simulink model "BPM_HA_Spin_sfun_16k"  (R2018a)
settings: configuration reference "ModelConfig_var" (kept outside this file)
InitFcn:
  | %% BUS initialization
  | Xabc.A = 0;
  | Xabc.B = 0;
  | Xabc.C = 0;
  | % -------------------------------------------------------------------------
  | Simulink.Bus.createObject(Xabc)
  | XabcBus = slBus1;
  | clear slBus1
  | 
  | %% Parameter Structure initialization
  | Motor_prm_init_bpm;
model workspace (MAT data in the model file):
  Mech_HAs_CF = 0
  Mech_HAs_J_drum = 0
  Mech_HAs_TR = 0
  Mech_HAs_damp = 0
  Mech_HAs_m_unb = 0
  Mech_HAs_r_unb = 0
  Mech_VAa_J_basket = 0
  Mech_VAa_J_impeller = 0
  Mech_VAa_basket_dens = 0
  Mech_VAa_basket_dia = 0
  Mech_VAa_belt_ratio = 0
  Mech_VAa_clothes_mass = 0
  Mech_VAa_gear_ratio = 0
  Mech_VAa_imp_dens = 0
  Mech_VAa_water_vol = 0
  Mech_VAs_D_r = 0
  Mech_VAs_I_zt = 0
  Mech_VAs_K = 2700
  Mech_VAs_T_f = 0
  Mech_VAs_belt_rat = 0
  Mech_VAs_d = 0
  Mech_VAs_e = 0
  Mech_VAs_m_b1 = 0
  Mech_VAs_m_b2 = 0
  Mech_VAs_m_d = 0
  Mech_VAs_m_t = 0
  Mech_VAs_m_u = 0
  Time_step = 6.25e-05
  bpm_B = 0
  bpm_Ipk = [0 1 2 3 4 5 6 7]
  bpm_Jrotor = 0
  bpm_Ld_0 = 0.02117
  bpm_Ld_a = [0.02117 0.02117 0.02117 0.02117 0.02117 0.02117 0.02117 0.02117]
  bpm_Ldq_sat_flag = 0
  bpm_Loss_Power = [0 1 2 3 4 5 6 7]
  bpm_Loss_Speed = [0 1 2 3 4 5 6 7]
  bpm_Loss_flag = 0
  bpm_Loss_th = 5
  bpm_Lq_0 = 0.02117
  bpm_Lq_b = [0.02117 0.02117 0.02117 0.02117 0.02117 0.02117 0.02117 0.02117]
  bpm_NPP = 0
  bpm_PM_flux_h1_0 = 0
  bpm_PM_rotor_alpha = 0
  bpm_Rs_0 = 0
  bpm_Rs_stator_alpha = 0
  bpm_TR = 1
  bpm_Temp_rotor_0 = 0
  bpm_Temp_stator_0 = 0
libraries: bpm_dq_S_noH_D_RL_HA_Spin_16k x1
settings Model: ParameterArgumentNames=Mech_HAs_CF,Mech_HAs_J_drum,Mech_HAs_TR,Mech_HAs_damp,Mech_HAs_m_unb,Mech_HAs_r_unb,Mech_VAa_J_basket,Mech_VAa_J_impeller,Mech_VAa_basket_dens,Mech_VAa_basket_dia,Mech_VAa_belt_ratio,Mech_VAa_clothes_mass,Mech_VAa_gear_ratio,Mech_VAa_imp_dens,Mech_VAa_water_vol,Mech_VAs_D_r,Mech_VAs_I_zt,Mech_VAs_K,Mech_VAs_T_f,Mech_VAs_belt_rat,Mech_VAs_d,Mech_VAs_e,Mech_VAs_m_b1,Mech_VAs_m_b2,Mech_VAs_m_d,Mech_VAs_m_t,Mech_VAs_m_u,Time_step,bpm_B,bpm_Ipk,bpm_Jrotor,bpm_Ld_0,bpm_Ld_a,bpm_Ldq_sat_flag,bpm_Loss_Power,bpm_Loss_Speed,bpm_Loss_flag,bpm_Loss_th,bpm_Lq_0,bpm_Lq_b,bpm_NPP,bpm_PM_flux_h1_0,bpm_PM_rotor_alpha,bpm_Rs_0,bpm_Rs_stator_alpha,bpm_TR,bpm_Temp_rotor_0,bpm_Temp_stator_0  OrderedModelArguments=off  Creator=BEDNASA  LastModifiedBy=BEDNASA
settings ConfigSetRef: SourceLocation=Base Workspace

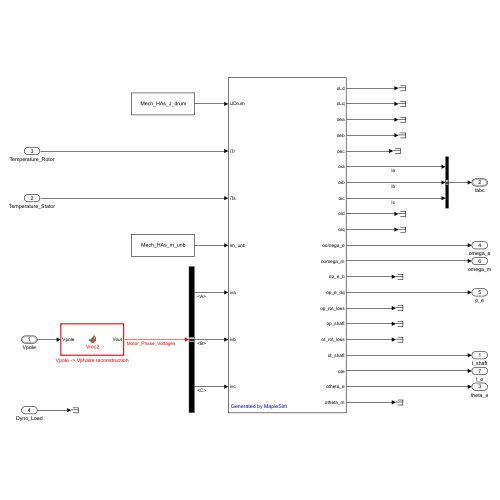
[thumbnail: Simulink's stored preview of the top-level diagram]
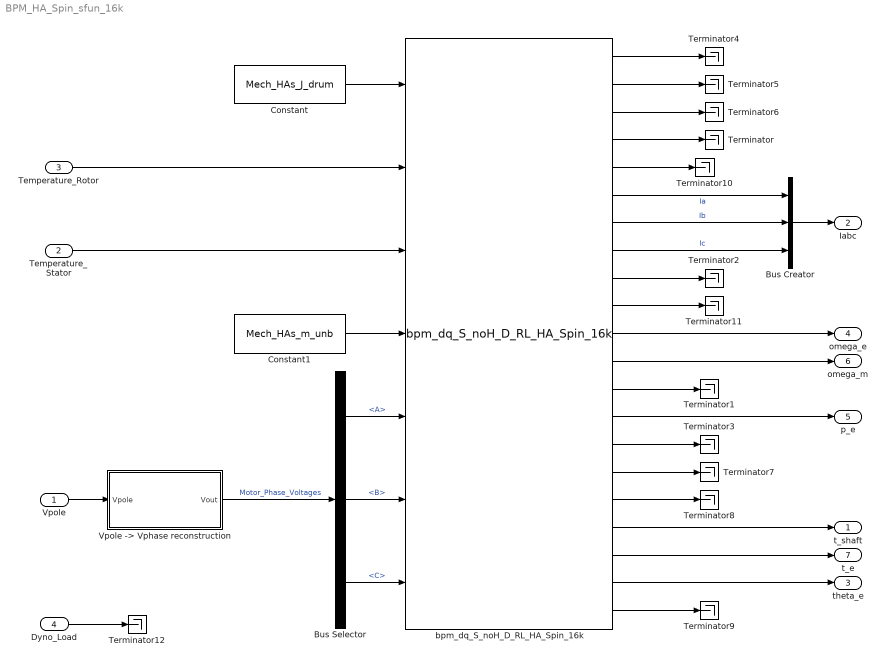
== system BPM_HA_Spin_sfun_16k ==
  Vpole : Inport  OutDataTypeStr=Bus: XabcBus
  Temperature_Stator : Inport  Port=2
  Temperature_Rotor : Inport  Port=3
  Dyno_Load : Inport  Port=4
  Bus Creator : BusCreator  Inputs=3
  Bus Selector : BusSelector  OutputSignals=A,B,C
  Constant : Constant  Value=Mech_HAs_J_drum
  Constant1 : Constant  Value=Mech_HAs_m_unb
  Terminator{,1..12} (13 alike) : Terminator
  "Vpole -> Vphase reconstruction" : MATLAB Function  TreatAsAtomicUnit=on
  bpm_dq_S_noH_D_RL_HA_Spin_16k : bpm_dq_S_noH_D_RL_HA_Spin_16k/bpm_dq_S_noH_D_RL_HA_Spin_16k  Description=Subsystem: bpm_dq_S_noH_D_RL_HA_Spin_16k  ic=[0., 0., 0., 0., 0.]  Par1=bpm_B  Par2=bpm_Ipk(1)  Par3=bpm_Ipk(2)  Par4=bpm_Ipk(3)  Par5=bpm_Ipk(4)  Par6=bpm_Ipk(5)  Par7=bpm_Ipk(6)  Par8=bpm_Ipk(7)  Par9=bpm_Ipk(8)  Par10=bpm_Jrotor  Par11=bpm_Ld_0  Par12=bpm_Ld_a(1)  Par13=bpm_Ld_a(2)  Par14=bpm_Ld_a(3)  Par15=bpm_Ld_a(4)  Par16=bpm_Ld_a(5)  Par17=bpm_Ld_a(6)  Par18=bpm_Ld_a(7)  Par19=bpm_Ld_a(8)  Par20=bpm_Lq_0  Par21=bpm_Lq_b(1)  Par22=bpm_Lq_b(2)  Par23=bpm_Lq_b(3)  Par24=bpm_Lq_b(4)  Par25=bpm_Lq_b(5)  Par26=bpm_Lq_b(6)  Par27=bpm_Lq_b(7)  Par28=bpm_Lq_b(8)  Par29=bpm_NPP  Par30=bpm_Loss_Power(1)  Par31=bpm_Loss_Power(2)  Par32=bpm_Loss_Power(3)  Par33=bpm_Loss_Power(4)  Par34=bpm_Loss_Power(5)  Par35=bpm_Loss_Power(6)  Par36=bpm_Loss_Power(7)  Par37=bpm_Loss_Power(8)  Par38=bpm_Loss_Speed(1)  Par39=bpm_Loss_Speed(2)  Par40=bpm_Loss_Speed(3)  Par41=bpm_Loss_Speed(4)  Par42=bpm_Loss_Speed(5)  Par43=bpm_Loss_Speed(6)  Par44=bpm_Loss_Speed(7)  Par45=bpm_Loss_Speed(8)  Par46=bpm_Loss_flag  Par47=bpm_Loss_th  Par48=bpm_Rs_0  Par49=bpm_Temp_rotor_0  Par50=bpm_Temp_stator_0  Par51=Time_step  Par52=bpm_Rs_stator_alpha  Par53=bpm_PM_rotor_alpha  Par54=bpm_PM_flux_h1_0  Par55=Mech_HAs_CF  Par56=Mech_HAs_TR  Par57=Mech_HAs_damp  Par58=0.  Par59=0.  Par60=0.  Par61=-9.8  Par62=-1.  Par63=Mech_HAs_r_unb  MinStep=1/40
  t_shaft : Outport  VectorParamsAs1DForOutWhenUnconnected=off
  Iabc : Outport  Port=2  OutDataTypeStr=Bus: XabcBus  VectorParamsAs1DForOutWhenUnconnected=off
  theta_e : Outport  Port=3  VectorParamsAs1DForOutWhenUnconnected=off
  omega_e : Outport  Port=4  VectorParamsAs1DForOutWhenUnconnected=off
  p_e : Outport  Port=5  VectorParamsAs1DForOutWhenUnconnected=off
  omega_m : Outport  Port=6  VectorParamsAs1DForOutWhenUnconnected=off
  t_e : Outport  Port=7  VectorParamsAs1DForOutWhenUnconnected=off
  wires:
  bpm_dq_S_noH_D_RL_HA_Spin_16k/4 -> Terminator/1
  bpm_dq_S_noH_D_RL_HA_Spin_16k/13 -> Terminator1/1
  bpm_dq_S_noH_D_RL_HA_Spin_16k/9 -> Terminator2/1
  bpm_dq_S_noH_D_RL_HA_Spin_16k/15 -> Terminator3/1
  bpm_dq_S_noH_D_RL_HA_Spin_16k/1 -> Terminator4/1
  bpm_dq_S_noH_D_RL_HA_Spin_16k/12 -> omega_m/1
  bpm_dq_S_noH_D_RL_HA_Spin_16k/11 -> omega_e/1
  bpm_dq_S_noH_D_RL_HA_Spin_16k/20 -> theta_e/1
  bpm_dq_S_noH_D_RL_HA_Spin_16k/19 -> t_e/1
  bpm_dq_S_noH_D_RL_HA_Spin_16k/18 -> t_shaft/1
  bpm_dq_S_noH_D_RL_HA_Spin_16k/2 -> Terminator5/1
  bpm_dq_S_noH_D_RL_HA_Spin_16k/3 -> Terminator6/1
  bpm_dq_S_noH_D_RL_HA_Spin_16k/16 -> Terminator7/1
  bpm_dq_S_noH_D_RL_HA_Spin_16k/14 -> p_e/1
  bpm_dq_S_noH_D_RL_HA_Spin_16k/17 -> Terminator8/1
  bpm_dq_S_noH_D_RL_HA_Spin_16k/10 -> Terminator11/1
  Bus Selector/3 -> bpm_dq_S_noH_D_RL_HA_Spin_16k/7  "<C>"
  Bus Selector/1 -> bpm_dq_S_noH_D_RL_HA_Spin_16k/5  "<A>"
  Bus Selector/2 -> bpm_dq_S_noH_D_RL_HA_Spin_16k/6  "<B>"
  "Vpole -> Vphase reconstruction"/1(Vout) -> Bus Selector/1  "Motor_Phase_Voltages"
  Vpole/1 -> "Vpole -> Vphase reconstruction"/1(Vpole)
  Dyno_Load/1 -> Terminator12/1
  bpm_dq_S_noH_D_RL_HA_Spin_16k/7 -> Bus Creator/2  "Ib"
  Bus Creator/1 -> Iabc/1
  bpm_dq_S_noH_D_RL_HA_Spin_16k/6 -> Bus Creator/1  "Ia"
  bpm_dq_S_noH_D_RL_HA_Spin_16k/8 -> Bus Creator/3  "Ic"
  Temperature_Rotor/1 -> bpm_dq_S_noH_D_RL_HA_Spin_16k/2
  Temperature_Stator/1 -> bpm_dq_S_noH_D_RL_HA_Spin_16k/3
  bpm_dq_S_noH_D_RL_HA_Spin_16k/21 -> Terminator9/1
  bpm_dq_S_noH_D_RL_HA_Spin_16k/5 -> Terminator10/1
  Constant/1 -> bpm_dq_S_noH_D_RL_HA_Spin_16k/1
  Constant1/1 -> bpm_dq_S_noH_D_RL_HA_Spin_16k/4

== matlab function BPM_HA_Spin_sfun_16k/Vpole -> Vphase reconstruction ==
  data: Vpole input Bus: XabcBus size=1; Vout output Bus: XabcBus
function Vout   = Vrec2(Vpole)

Va = Vpole.A;
Vb = Vpole.B;
Vc = Vpole.C;

Vn = (Va + Vb + Vc)/3;

Vphase.A = Va - Vn;
Vphase.B = Vb - Vn;
Vphase.C = Vc - Vn;

Vline.A = Va - Vb;  % Vab
Vline.B = Vb - Vc;  % Vbc
Vline.C = Vc - Va;  % Vca

Vout = Vphase;
end
